simulink model "PMSM_FOC_ClosedLoop"  (R2025b)
settings: Solver=ode3  StartTime=0.0  StopTime=0.4  FixedStep=Ts_sim  RelTol=1e-3
PreLoadFcn:
  | params_pmsm_inverter
undefined symbols (not defined in the file or in its folder): Iq_max, J, Ki_curr, Ki_spd, Kp_curr, Kp_spd, Ld, Lq, pp, PsiPM, Rs, Ts_ctrl, Vdc, Vph_max
libraries: nesl_utility x13, fl_lib x9, ee_lib x8, slpidlib x3, simulink x2
(part 1 of 2)
settings Model: Creator=Harish  LastModifiedBy=Harish

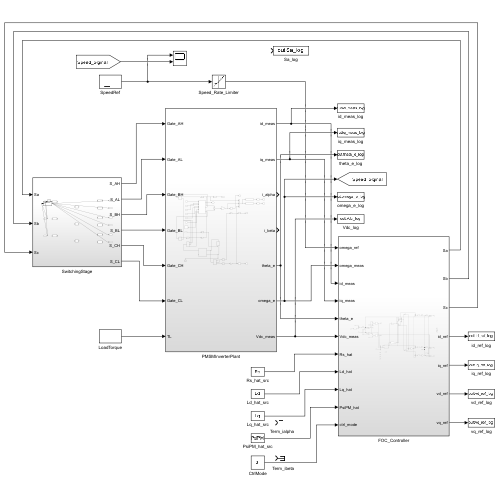
[thumbnail: Simulink's stored preview of the top-level diagram]
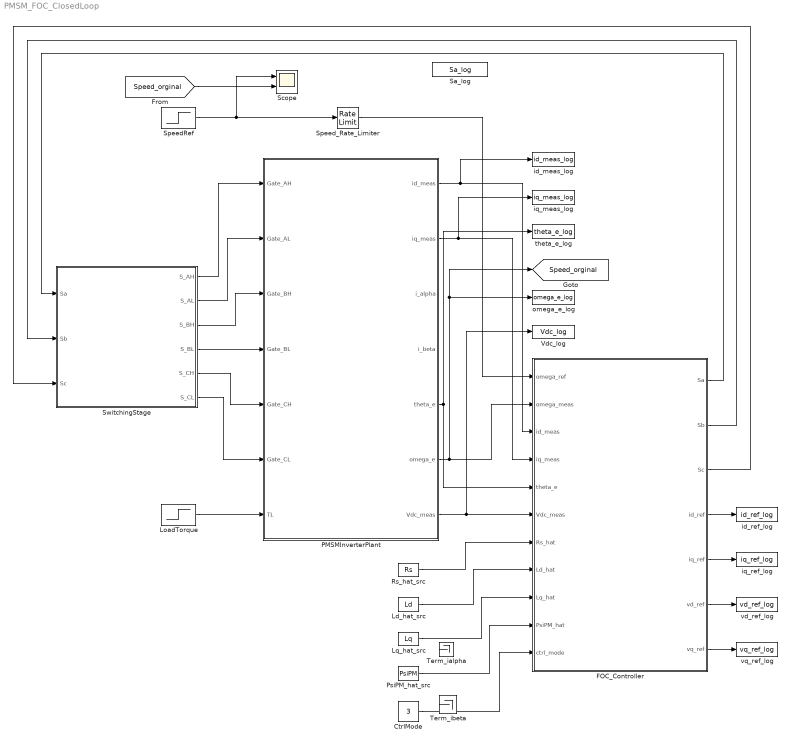
== system PMSM_FOC_ClosedLoop ==
  CtrlMode : Constant  Value=3
  FOC_Controller : Subsystem
  Ld_hat_src : Constant  Value=Ld
  LoadTorque : Step  Time=0.25  Before=0.0  After=0.05  SampleTime=0
  Lq_hat_src : Constant  Value=Lq
  PMSMInverterPlant : Subsystem
  PsiPM_hat_src : Constant  Value=PsiPM
  Rs_hat_src : Constant  Value=Rs
  Sa_log : ToWorkspace  VariableName=Sa_log  SaveFormat=Timeseries  SampleTime=-1
  Scope : Scope  NumInputPorts=2
      settings: ActiveDisplayYMinimum=-24.999999999999993  ActiveDisplayYMaximum=225
  SpeedRef : Step  Time=0.05  After=200  SampleTime=Ts_ctrl
  Speed_Rate_Limiter : RateLimiter  RisingSlewLimit=inf  FallingSlewLimit=-inf  SampleTimeMode=inherited
  SwitchingStage : Subsystem
  Term_ialpha : Terminator
  Term_ibeta : Terminator
  Vdc_log : ToWorkspace  VariableName=Vdc_log  SaveFormat=Timeseries  SampleTime=-1
  id_meas_log : ToWorkspace  VariableName=id_meas_log  SaveFormat=Timeseries  SampleTime=-1
  id_ref_log : ToWorkspace  VariableName=id_ref_log  SaveFormat=Timeseries  SampleTime=-1
  iq_meas_log : ToWorkspace  VariableName=iq_meas_log  SaveFormat=Timeseries  SampleTime=-1
  iq_ref_log : ToWorkspace  VariableName=iq_ref_log  SaveFormat=Timeseries  SampleTime=-1
  omega_e_log : ToWorkspace  VariableName=omega_e_log  SaveFormat=Timeseries  SampleTime=-1
  theta_e_log : ToWorkspace  VariableName=theta_e_log  SaveFormat=Timeseries  SampleTime=-1
  vd_ref_log : ToWorkspace  VariableName=vd_ref_log  SaveFormat=Timeseries  SampleTime=-1
  vq_ref_log : ToWorkspace  VariableName=vq_ref_log  SaveFormat=Timeseries  SampleTime=-1
  tag scope: Speed_orginal=global
  wires:
  [Speed_orginal] -> Scope/2
  SwitchingStage/5(S_CH) -> PMSMInverterPlant/5(Gate_CH)
  SwitchingStage/1(S_AH) -> PMSMInverterPlant/1(Gate_AH)
  SpeedRef/1 -> Scope/1, Speed_Rate_Limiter/1
  SwitchingStage/6(S_CL) -> PMSMInverterPlant/6(Gate_CL)
  FOC_Controller/2(Sb) -> SwitchingStage/2(Sb)
  PMSMInverterPlant/7(Vdc_meas) -> Vdc_log/1, FOC_Controller/6(Vdc_meas)
  SwitchingStage/2(S_AL) -> PMSMInverterPlant/2(Gate_AL)
  SwitchingStage/3(S_BH) -> PMSMInverterPlant/3(Gate_BH)
  PMSMInverterPlant/1(id_meas) -> FOC_Controller/3(id_meas), id_meas_log/1
  SwitchingStage/4(S_BL) -> PMSMInverterPlant/4(Gate_BL)
  LoadTorque/1 -> PMSMInverterPlant/7(TL)
  Speed_Rate_Limiter/1 -> FOC_Controller/1(omega_ref)
  FOC_Controller/3(Sc) -> SwitchingStage/3(Sc)
  PMSMInverterPlant/2(iq_meas) -> FOC_Controller/4(iq_meas), iq_meas_log/1
  PMSMInverterPlant/5(theta_e) -> FOC_Controller/5(theta_e), theta_e_log/1
  PMSMInverterPlant/6(omega_e) -> [Speed_orginal], omega_e_log/1, FOC_Controller/2(omega_meas)
  Rs_hat_src/1 -> FOC_Controller/7(Rs_hat)
  Ld_hat_src/1 -> FOC_Controller/8(Ld_hat)
  Lq_hat_src/1 -> FOC_Controller/9(Lq_hat)
  PsiPM_hat_src/1 -> FOC_Controller/10(PsiPM_hat)
  CtrlMode/1 -> FOC_Controller/11(ctrl_mode)
  FOC_Controller/1(Sa) -> SwitchingStage/1(Sa)
  FOC_Controller/4(id_ref) -> id_ref_log/1
  FOC_Controller/5(iq_ref) -> iq_ref_log/1
  FOC_Controller/6(vd_ref) -> vd_ref_log/1
  FOC_Controller/7(vq_ref) -> vq_ref_log/1

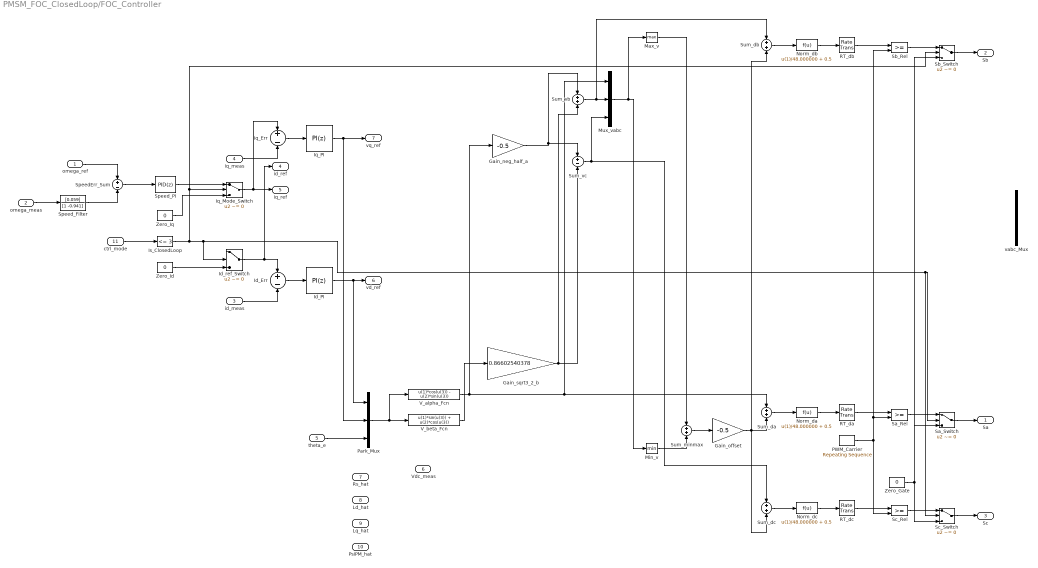
== system PMSM_FOC_ClosedLoop/FOC_Controller ==
  omega_ref : Inport  SampleTime=Ts_ctrl
  omega_meas : Inport  Port=2  SampleTime=Ts_ctrl
  id_meas : Inport  Port=3  SampleTime=Ts_ctrl
  iq_meas : Inport  Port=4  SampleTime=Ts_ctrl
  theta_e : Inport  Port=5  SampleTime=Ts_ctrl
  Vdc_meas : Inport  Port=6  SampleTime=Ts_ctrl
  Rs_hat : Inport  Port=7  SampleTime=Ts_ctrl
  Ld_hat : Inport  Port=8  SampleTime=Ts_ctrl
  Lq_hat : Inport  Port=9  SampleTime=Ts_ctrl
  PsiPM_hat : Inport  Port=10  SampleTime=Ts_ctrl
  ctrl_mode : Inport  Port=11  SampleTime=Ts_ctrl
  Gain_neg_half_a : Gain  Gain=-0.5
  Gain_offset : Gain  Gain=-0.5
  Gain_sqrt3_2_b : Gain  Gain=0.86602540378
  Id_Err : Sum  Inputs=+-
  Id_PI : slpidlib/PID Controller  Controller=PI  Form=Parallel  TimeDomain=Discrete-time  UseExternalTs=off  SampleTime=Ts_ctrl  IntegratorMethod=Forward Euler  FilterMethod=Forward Euler  ControllerParametersSource=internal  P=Kp_curr  I=Ki_curr  UseKiTs=off  D=0  UseExternalDerivativeSource=off  N=100  UseFilter=on  TunerSelectOption=Transfer Function Based (PID Tuner App)  InitialConditionSource=internal  InitialConditionForIntegrator=0  InitialConditionForFilter=0  DifferentiatorICPrevScaledInput=0  ExternalReset=none  TrackingMode=off  Kt=1  LimitOutput=on  SatLimitsSource=internal  UpperSaturationLimit=Vph_max  LowerSaturationLimit=-Vph_max  LinearizeAsGain=off  AntiWindupMode=clamping  Kb=1  LimitIntegrator=off  UpperIntegratorSaturationLimit=inf  LowerIntegratorSaturationLimit=-inf  POutMin=[]  POutMax=[]  IOutMin=[]  IOutMax=[]  DOutMin=[]  DOutMax=[]  NOutMin=[]  NOutMax=[]  SumOutMin=[]  SumOutMax=[]  SaturationOutMin=[]  SaturationOutMax=[]  PParamMin=[]  PParamMax=[]  IParamMin=[]  IParamMax=[]  DParamMin=[]  DParamMax=[]  NParamMin=[]  NParamMax=[]  KbParamMin=[]  KbParamMax=[]  KtParamMin=[]  KtParamMax=[]  KbOutMin=[]  KbOutMax=[]  KtOutMin=[]  KtOutMax=[]  IntegratorOutMin=[]  IntegratorOutMax=[]  FilterOutMin=[]  FilterOutMax=[]  SumI1OutMin=[]  SumI1OutMax=[]  SumI2OutMin=[]  SumI2OutMax=[]  SumI3OutMin=[]  SumI3OutMax=[]  SumI4OutMin=[]  SumI4OutMax=[]  SumDOutMin=[]  SumDOutMax=[]  DifferentiatorOutMin=[]  DifferentiatorOutMax=[]  FilterDiffOutCoefMin=[]  FilterDiffOutCoefMax=[]  ReciprocalOutMin=[]  ReciprocalOutMax=[]  SumDenOutMin=[]  SumDenOutMax=[]  SumNumOutMin=[]  SumNumOutMax=[]  DivideOutMin=[]  DivideOutMax=[]  UdiffTsProdOutMin=[]  UdiffTsProdOutMax=[]  NTsProdOutMin=[]  NTsProdOutMax=[]  UintegralTsProdOutMin=[]  UintegralTsProdOutMax=[]  UngainTsProdOutMin=[]  UngainTsProdOutMax=[]  ClampingZeroOutDataTypeStr=Inherit: Inherit via back propagation  ClampingZeroOutMin=[]  ClampingZeroOutMax=[]  FilterDenConstantOutDataTypeStr=Inherit: Inherit via back propagation  FilterDenConstantOutMin=[]  FilterDenConstantOutMax=[]  PCopyOutDataTypeStr=Inherit: Inherit via back propagation  PCopyOutMin=[]  PCopyOutMax=[]  NCopyOutDataTypeStr=Inherit: Inherit via back propagation  NCopyOutMin=[]  NCopyOutMax=[]  IntegratorContinuousStateAttributes=''  IntegratorStateMustResolveToSignalObject=off  IntegratorRTWStateStorageClass=Auto  FilterContinuousStateAttributes=''  FilterStateMustResolveToSignalObject=off  FilterRTWStateStorageClass=Auto  ParallelPVariant=InternalParameters  IdealPVariant=Disabled  IVariant=InternalParameters  DVariant=Disabled  IntegratorVariant=Discrete  SatVariant=Enabled  AWVariant=DiscClampingParallel  PCopyVariant=Disabled  TRVariant=Disabled  FdbkBlocksVariant=Forward  IdealPFdbkVariant=Disabled  SatFdbkVariant=Disabled  DerivativeFilterVariant=Disabled  NVariant=Disabled  NCopyVariant=Disabled_SignalSpec  FilterICVariant=Disabled  IntegratorICVariant=InternalICs  ExternalResetVariant=Disabled  TRSumVariant=Passthrough  SumFdbkVariant=Disabled  SumVariant=Sum_PI  TsampFilterVariant=InternalTs  TsampNgainVariant=Passthrough  TsampIntegralVariant=Disabled_SignalSpec  ExternalSaturationOutDataTypeStr=Inherit: Same as second input  DerivativeSourceVariant=Disabled  PreIntVariant=InternalPreInt
      settings: LibrarySourceBlock=simulink/Discrete/Discrete PID Controller
  Id_ref_Switch : Switch  Criteria=u2 ~= 0  SaturateOnIntegerOverflow=off  InputSameDT=off
  Iq_Err : Sum  Inputs=+-
  Iq_Mode_Switch : Switch  Criteria=u2 ~= 0  SaturateOnIntegerOverflow=off  InputSameDT=off
  Iq_PI : slpidlib/PID Controller  Controller=PI  Form=Parallel  TimeDomain=Discrete-time  UseExternalTs=off  SampleTime=Ts_ctrl  IntegratorMethod=Forward Euler  FilterMethod=Forward Euler  ControllerParametersSource=internal  P=Kp_curr  I=Ki_curr  UseKiTs=off  D=0  UseExternalDerivativeSource=off  N=100  UseFilter=on  TunerSelectOption=Transfer Function Based (PID Tuner App)  InitialConditionSource=internal  InitialConditionForIntegrator=0  InitialConditionForFilter=0  DifferentiatorICPrevScaledInput=0  ExternalReset=none  TrackingMode=off  Kt=1  LimitOutput=on  SatLimitsSource=internal  UpperSaturationLimit=Vph_max  LowerSaturationLimit=-Vph_max  LinearizeAsGain=off  AntiWindupMode=clamping  Kb=1  LimitIntegrator=off  UpperIntegratorSaturationLimit=inf  LowerIntegratorSaturationLimit=-inf  POutMin=[]  POutMax=[]  IOutMin=[]  IOutMax=[]  DOutMin=[]  DOutMax=[]  NOutMin=[]  NOutMax=[]  SumOutMin=[]  SumOutMax=[]  SaturationOutMin=[]  SaturationOutMax=[]  PParamMin=[]  PParamMax=[]  IParamMin=[]  IParamMax=[]  DParamMin=[]  DParamMax=[]  NParamMin=[]  NParamMax=[]  KbParamMin=[]  KbParamMax=[]  KtParamMin=[]  KtParamMax=[]  KbOutMin=[]  KbOutMax=[]  KtOutMin=[]  KtOutMax=[]  IntegratorOutMin=[]  IntegratorOutMax=[]  FilterOutMin=[]  FilterOutMax=[]  SumI1OutMin=[]  SumI1OutMax=[]  SumI2OutMin=[]  SumI2OutMax=[]  SumI3OutMin=[]  SumI3OutMax=[]  SumI4OutMin=[]  SumI4OutMax=[]  SumDOutMin=[]  SumDOutMax=[]  DifferentiatorOutMin=[]  DifferentiatorOutMax=[]  FilterDiffOutCoefMin=[]  FilterDiffOutCoefMax=[]  ReciprocalOutMin=[]  ReciprocalOutMax=[]  SumDenOutMin=[]  SumDenOutMax=[]  SumNumOutMin=[]  SumNumOutMax=[]  DivideOutMin=[]  DivideOutMax=[]  UdiffTsProdOutMin=[]  UdiffTsProdOutMax=[]  NTsProdOutMin=[]  NTsProdOutMax=[]  UintegralTsProdOutMin=[]  UintegralTsProdOutMax=[]  UngainTsProdOutMin=[]  UngainTsProdOutMax=[]  ClampingZeroOutDataTypeStr=Inherit: Inherit via back propagation  ClampingZeroOutMin=[]  ClampingZeroOutMax=[]  FilterDenConstantOutDataTypeStr=Inherit: Inherit via back propagation  FilterDenConstantOutMin=[]  FilterDenConstantOutMax=[]  PCopyOutDataTypeStr=Inherit: Inherit via back propagation  PCopyOutMin=[]  PCopyOutMax=[]  NCopyOutDataTypeStr=Inherit: Inherit via back propagation  NCopyOutMin=[]  NCopyOutMax=[]  IntegratorContinuousStateAttributes=''  IntegratorStateMustResolveToSignalObject=off  IntegratorRTWStateStorageClass=Auto  FilterContinuousStateAttributes=''  FilterStateMustResolveToSignalObject=off  FilterRTWStateStorageClass=Auto  ParallelPVariant=InternalParameters  IdealPVariant=Disabled  IVariant=InternalParameters  DVariant=Disabled  IntegratorVariant=Discrete  SatVariant=Enabled  AWVariant=DiscClampingParallel  PCopyVariant=Disabled  TRVariant=Disabled  FdbkBlocksVariant=Forward  IdealPFdbkVariant=Disabled  SatFdbkVariant=Disabled  DerivativeFilterVariant=Disabled  NVariant=Disabled  NCopyVariant=Disabled_SignalSpec  FilterICVariant=Disabled  IntegratorICVariant=InternalICs  ExternalResetVariant=Disabled  TRSumVariant=Passthrough  SumFdbkVariant=Disabled  SumVariant=Sum_PI  TsampFilterVariant=InternalTs  TsampNgainVariant=Passthrough  TsampIntegralVariant=Disabled_SignalSpec  ExternalSaturationOutDataTypeStr=Inherit: Same as second input  DerivativeSourceVariant=Disabled  PreIntVariant=InternalPreInt
      settings: LibrarySourceBlock=simulink/Discrete/Discrete PID Controller
  Is_ClosedLoop : simulink/Logic and Bit Operations/Compare To Constant  relop=<=  const=3  OutDataTypeStr=boolean
  Max_v : MinMax  Function=max
  Min_v : MinMax
  Mux_vabc : Mux  Inputs=3
  Norm_da : Fcn  Expr=u(1)/48.000000 + 0.5
  Norm_db : Fcn  Expr=u(1)/48.000000 + 0.5
  Norm_dc : Fcn  Expr=u(1)/48.000000 + 0.5
  PWM_Carrier : simulink/Sources/Repeating Sequence  rep_seq_t=[0, Ts_ctrl/2, Ts_ctrl]  rep_seq_y=[0, 1, 0]
  Park_Mux : Mux  Inputs=3
  RT_da : RateTransition  OutPortSampleTime=Ts_sim
  RT_db : RateTransition  OutPortSampleTime=Ts_sim
  RT_dc : RateTransition  OutPortSampleTime=Ts_sim
  Sa_Rel : RelationalOperator  OutDataTypeStr=boolean  RndMeth=Simplest  InputSameDT=off
  Sa_Switch : Switch  Criteria=u2 ~= 0  SaturateOnIntegerOverflow=off  InputSameDT=off
  Sb_Rel : RelationalOperator  OutDataTypeStr=boolean  RndMeth=Simplest  InputSameDT=off
  Sb_Switch : Switch  Criteria=u2 ~= 0  SaturateOnIntegerOverflow=off  InputSameDT=off
  Sc_Rel : RelationalOperator  OutDataTypeStr=boolean  RndMeth=Simplest  InputSameDT=off
  Sc_Switch : Switch  Criteria=u2 ~= 0  SaturateOnIntegerOverflow=off  InputSameDT=off
  SpeedErr_Sum : Sum  Inputs=+-
  Speed_Filter : DiscreteFilter  Numerator=[0.059]  Denominator=[1 -0.941]  SampleTime=Ts_ctrl
  Speed_PI : slpidlib/PID Controller  Controller=PID  Form=Parallel  TimeDomain=Discrete-time  UseExternalTs=off  SampleTime=Ts_ctrl  IntegratorMethod=Forward Euler  FilterMethod=Forward Euler  ControllerParametersSource=internal  P=Kp_spd  I=Ki_spd  UseKiTs=off  D=0  UseExternalDerivativeSource=off  N=100  UseFilter=on  TunerSelectOption=Transfer Function Based (PID Tuner App)  InitialConditionSource=internal  InitialConditionForIntegrator=0  InitialConditionForFilter=0  DifferentiatorICPrevScaledInput=0  ExternalReset=none  TrackingMode=off  Kt=1  LimitOutput=on  SatLimitsSource=internal  UpperSaturationLimit=Iq_max  LowerSaturationLimit=-Iq_max  LinearizeAsGain=on  AntiWindupMode=clamping  Kb=1  LimitIntegrator=off  UpperIntegratorSaturationLimit=inf  LowerIntegratorSaturationLimit=-inf  POutMin=[]  POutMax=[]  IOutMin=[]  IOutMax=[]  DOutMin=[]  DOutMax=[]  NOutMin=[]  NOutMax=[]  SumOutMin=[]  SumOutMax=[]  SaturationOutMin=[]  SaturationOutMax=[]  PParamMin=[]  PParamMax=[]  IParamMin=[]  IParamMax=[]  DParamMin=[]  DParamMax=[]  NParamMin=[]  NParamMax=[]  KbParamMin=[]  KbParamMax=[]  KtParamMin=[]  KtParamMax=[]  KbOutMin=[]  KbOutMax=[]  KtOutMin=[]  KtOutMax=[]  IntegratorOutMin=[]  IntegratorOutMax=[]  FilterOutMin=[]  FilterOutMax=[]  SumI1OutMin=[]  SumI1OutMax=[]  SumI2OutMin=[]  SumI2OutMax=[]  SumI3OutMin=[]  SumI3OutMax=[]  SumI4OutMin=[]  SumI4OutMax=[]  SumDOutMin=[]  SumDOutMax=[]  DifferentiatorOutMin=[]  DifferentiatorOutMax=[]  FilterDiffOutCoefMin=[]  FilterDiffOutCoefMax=[]  ReciprocalOutMin=[]  ReciprocalOutMax=[]  SumDenOutMin=[]  SumDenOutMax=[]  SumNumOutMin=[]  SumNumOutMax=[]  DivideOutMin=[]  DivideOutMax=[]  UdiffTsProdOutMin=[]  UdiffTsProdOutMax=[]  NTsProdOutMin=[]  NTsProdOutMax=[]  UintegralTsProdOutMin=[]  UintegralTsProdOutMax=[]  UngainTsProdOutMin=[]  UngainTsProdOutMax=[]  ClampingZeroOutDataTypeStr=Inherit: Inherit via back propagation  ClampingZeroOutMin=[]  ClampingZeroOutMax=[]  FilterDenConstantOutDataTypeStr=Inherit: Inherit via back propagation  FilterDenConstantOutMin=[]  FilterDenConstantOutMax=[]  PCopyOutDataTypeStr=Inherit: Inherit via back propagation  PCopyOutMin=[]  PCopyOutMax=[]  NCopyOutDataTypeStr=Inherit: Inherit via back propagation  NCopyOutMin=[]  NCopyOutMax=[]  IntegratorContinuousStateAttributes=''  IntegratorStateMustResolveToSignalObject=off  IntegratorRTWStateStorageClass=Auto  FilterContinuousStateAttributes=''  FilterStateMustResolveToSignalObject=off  FilterRTWStateStorageClass=Auto  ParallelPVariant=InternalParameters  IdealPVariant=Disabled  IVariant=InternalParameters  DVariant=InternalParameters  IntegratorVariant=Discrete  SatVariant=Enabled  AWVariant=DiscClampingParallel  PCopyVariant=Disabled  TRVariant=Disabled  FdbkBlocksVariant=Forward  IdealPFdbkVariant=Disabled  SatFdbkVariant=Disabled  DerivativeFilterVariant=ForwardEulerFilter  NVariant=InternalParameters  NCopyVariant=Disabled  FilterICVariant=InternalICsFilter  IntegratorICVariant=InternalICs  ExternalResetVariant=Disabled  TRSumVariant=Passthrough  SumFdbkVariant=Disabled  SumVariant=Sum_PID  TsampFilterVariant=InternalTs  TsampNgainVariant=Passthrough  TsampIntegralVariant=Disabled_SignalSpec  ExternalSaturationOutDataTypeStr=Inherit: Same as second input  DerivativeSourceVariant=ErrorSignal  PreIntVariant=InternalPreInt
  Sum_da : Sum
  Sum_db : Sum
  Sum_dc : Sum
  Sum_minmax : Sum
  Sum_vb : Sum
  Sum_vc : Sum  Inputs=+-
  V_alpha_Fcn : Fcn  Expr=u(1)*cos(u(3)) - u(2)*sin(u(3))
  V_beta_Fcn : Fcn  Expr=u(1)*sin(u(3)) + u(2)*cos(u(3))
  Zero_Gate : Constant  Value=0  OutDataTypeStr=boolean  SampleTime=Ts_ctrl
  Zero_Id : Constant  Value=0
  Zero_Iq : Constant  Value=0  SampleTime=Ts_ctrl
  vabc_Mux : Mux  Inputs=3
  Sa : Outport
  Sb : Outport  Port=2
  Sc : Outport  Port=3
  id_ref : Outport  Port=4  SampleTime=Ts_ctrl
  iq_ref : Outport  Port=5  SampleTime=Ts_ctrl
  vd_ref : Outport  Port=6  SampleTime=Ts_ctrl
  vq_ref : Outport  Port=7  SampleTime=Ts_ctrl
  wires:
  Speed_PI/1 -> Iq_Mode_Switch/1
  Zero_Id/1 -> Id_ref_Switch/3
  omega_meas/1 -> Speed_Filter/1
  Is_ClosedLoop/1 -> Sc_Switch/2, Sa_Switch/2, Id_ref_Switch/2, Iq_Mode_Switch/2, Sb_Switch/2
  ctrl_mode/1 -> Is_ClosedLoop/1
  Zero_Iq/1 -> Iq_Mode_Switch/3
  Id_Err/1 -> Id_PI/1
  omega_ref/1 -> SpeedErr_Sum/1
  Speed_Filter/1 -> SpeedErr_Sum/2
  Zero_Gate/1 -> Sb_Switch/3, Sc_Switch/3, Sa_Switch/3
  SpeedErr_Sum/1 -> Speed_PI/1
  iq_meas/1 -> Iq_Err/2
  Iq_Mode_Switch/1 -> Iq_Err/1, iq_ref/1
  theta_e/1 -> Park_Mux/3
  Id_ref_Switch/1 -> Id_Err/1, id_ref/1
  id_meas/1 -> Id_Err/2
  Iq_Err/1 -> Iq_PI/1
  Sb_Rel/1 -> Sb_Switch/1
  Sum_db/1 -> Norm_db/1
  Iq_PI/1 -> Park_Mux/2, vq_ref/1
  Sb_Switch/1 -> Sb/1
  Gain_neg_half_a/1 -> Sum_vc/1, Sum_vb/1
  Id_PI/1 -> Park_Mux/1, vd_ref/1
  Norm_dc/1 -> RT_dc/1
  Park_Mux/1 -> V_alpha_Fcn/1, V_beta_Fcn/1
  Sa_Switch/1 -> Sa/1
  Sum_da/1 -> Norm_da/1
  V_alpha_Fcn/1 -> Sum_da/1, Mux_vabc/1, Gain_neg_half_a/1
  Gain_offset/1 -> Sum_da/2, Sum_db/2, Sum_dc/2
  V_beta_Fcn/1 -> Gain_sqrt3_2_b/1
  Gain_sqrt3_2_b/1 -> Sum_vb/2, Sum_vc/2
  Min_v/1 -> Sum_minmax/2
  Sum_vb/1 -> Sum_db/1, Mux_vabc/2
  Sum_dc/1 -> Norm_dc/1
  Sum_vc/1 -> Sum_dc/1, Mux_vabc/3
  Mux_vabc/1 -> Max_v/1, Min_v/1
  Max_v/1 -> Sum_minmax/1
  Sum_minmax/1 -> Gain_offset/1
  Norm_db/1 -> RT_db/1
  Norm_da/1 -> RT_da/1
  RT_db/1 -> Sb_Rel/1
  RT_da/1 -> Sa_Rel/1
  PWM_Carrier/1 -> Sb_Rel/2, Sa_Rel/2, Sc_Rel/2
  Sc_Switch/1 -> Sc/1
  RT_dc/1 -> Sc_Rel/1
  Sa_Rel/1 -> Sa_Switch/1
  Sc_Rel/1 -> Sc_Switch/1

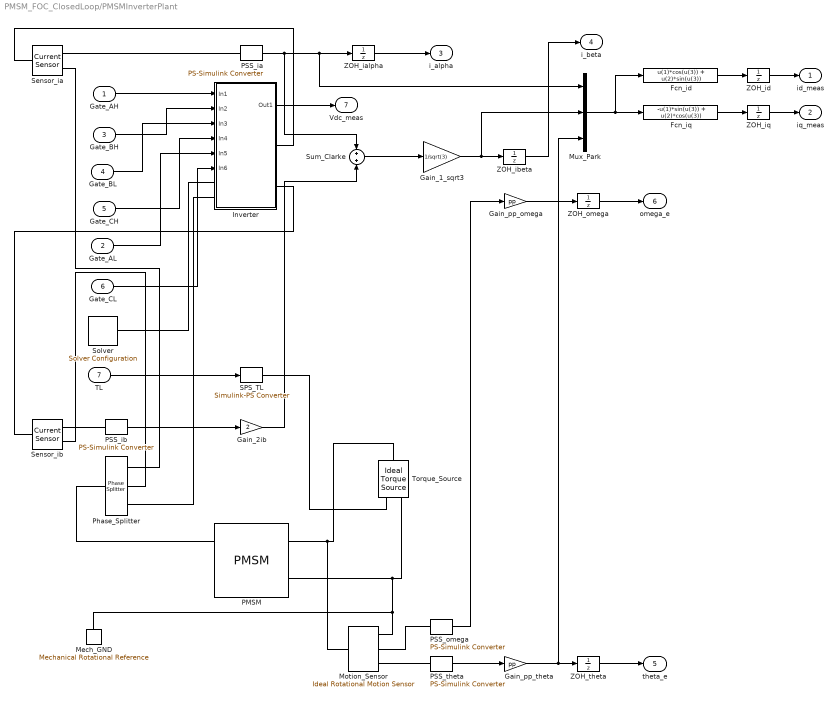
== system PMSM_FOC_ClosedLoop/PMSMInverterPlant ==
  Gate_AH : Inport
  Gate_AL : Inport  Port=2
  Gate_BH : Inport  Port=3
  Gate_BL : Inport  Port=4
  Gate_CH : Inport  Port=5
  Gate_CL : Inport  Port=6
  TL : Inport  Port=7
  Fcn_id : Fcn  Expr=u(1)*cos(u(3)) + u(2)*sin(u(3))
  Fcn_iq : Fcn  Expr=-u(1)*sin(u(3)) + u(2)*cos(u(3))
  Gain_1_sqrt3 : Gain  Gain=1/sqrt(3)
  Gain_2ib : Gain  Gain=2
  Gain_pp_omega : Gain  Gain=pp
  Gain_pp_theta : Gain  Gain=pp
  Inverter : Subsystem
  Mech_GND : fl_lib/Mechanical/Rotational Elements/Mechanical Rotational Reference
  Motion_Sensor : fl_lib/Mechanical/Mechanical Sensors/Ideal Rotational Motion Sensor  reference=foundation.enum.MeasurementReference.difference  acceleration_port=false  velocity_port=true  position_port=true  wrap_angle=false  offset=0 rad
  Mux_Park : Mux  Inputs=3
  PMSM : ee_lib/Electromechanical/Permanent Magnet/PMSM  port_option=1  winding_type=ee.enum.electromech.statorconfiguration.wye  machine_param=ee.enum.pmsm.parameterization.constant  nPolePairs=pp  pmflux_param=ee.enum.pmflux.fluxlinkage  pm_flux_linkage=PsiPM Wb  torque_constant=0.18 N*m/A  back_emf_constant=0.18 V*s/rad  stator_param=1  Ld=Ld H  Lq=Lq H  idVec=[-200, 0, 200] A  iqVec=[-200, 0, 200] A  LdMatrix=0.0002 * ones(3, 3) H  LqMatrix=0.0002 * ones(3, 3) H  PmMatrix=0.1 * ones(3, 3) Wb  ktMatrix=0.18 * ones(3, 3) N*m/A  keMatrix=0.18 * ones(3, 3) V*s/rad  L0=0.00016 H  Ls=0.0002 H  Lm=-0.00002 H  Ms=0.00002 H  Rs=Rs Ohm  zero_sequence=ee.enum.park.zerosequence.include  axes_param=ee.enum.rotorangle.daxis  loss_param=ee.enum.ironloss.none  losses_oc=[0, 0, 0] W  losses_sc=[0, 0, 0] W  f_losses=60 Hz  Isc_losses=95 A  J=J kg*m^2  lam=B_fric N*m*s/rad  i_d_specify=off  i_d_priority=None  i_d=0 A  i_d_nominal_specify=off  i_d_nominal_value=1  i_d_nominal_unit=A  i_q_specify=off  i_q_priority=None  i_q=0 A  i_q_nominal_specify=off  i_q_nominal_value=1  i_q_nominal_unit=A  torque_specify=off  torque_priority=None  torque=0 N*m  torque_nominal_specify=off  torque_nominal_value=1  torque_nominal_unit=N*m  angular_velocity_specify=off  angular_velocity_priority=High  angular_velocity=0 rpm  angular_velocity_nominal_specify=off  angular_velocity_nominal_value=1  angular_velocity_nominal_unit=rpm  angular_position_specify=off  angular_position_priority=High  angular_position=0 deg  angular_position_nominal_specify=off  angular_position_nominal_value=1  angular_position_nominal_unit=deg  alpha=3.93e-3 1/K  alpha_flux=-0.001 1/K  Tmeas=298.15 K  stator_thermal_mass=100 J/K  rotor_thermal_mass=200 J/K  Rm_percent_rotor=90  Rd_percent_rotor=30  temperatureA_specify=off  temperatureA_priority=High  temperatureA=25 degC  temperatureA_nominal_specify=off  temperatureA_nominal_value=1  temperatureA_nominal_unit=degC  temperatureB_specify=off  temperatureB_priority=High  temperatureB=25 degC  temperatureB_nominal_specify=off  temperatureB_nominal_value=1  temperatureB_nominal_unit=degC  temperatureC_specify=off  temperatureC_priority=High  temperatureC=25 degC  temperatureC_nominal_specify=off  temperatureC_nominal_value=1  temperatureC_nominal_unit=degC  temperatureR_specify=off  temperatureR_priority=High  temperatureR=25 degC  temperatureR_nominal_specify=off  temperatureR_nominal_value=1  temperatureR_nominal_unit=degC
      settings: InternalSimscapePortConfiguration="{\"Bottom\":[],\"Left\":[{\"id\":\"N\",\"label\":\"~\",\"type\":\"foundation.electrical.three_phase\"},{\"id\":\"n\",\"label\":\"n\",\"type\":\"foundation.electrical.electrical\"}],\"Right\":[{\"id\":\"R\",\"label\":\"R\",\"type\":\"foundation.mechanical.rotational.rotational\"},{\"id\":\"C\",\"label\":\"C\",\"type\":\"foundation.mechanical.rotational.rotational\"}],\"Top\":[]}"
  PSS_ia : nesl_utility/PS-Simulink Converter  PhysicalDomain=network_engine_domain  SubClassName=ps_output  LeftPortType=input  RightPortType=output  PseudoPeriodic=off  Frequencies=[]  VectorFormat=inherit  Unit=inherit  AffineConversion=off
  PSS_ib : nesl_utility/PS-Simulink Converter  PhysicalDomain=network_engine_domain  SubClassName=ps_output  LeftPortType=input  RightPortType=output  PseudoPeriodic=off  Frequencies=[]  VectorFormat=inherit  Unit=inherit  AffineConversion=off
  PSS_omega : nesl_utility/PS-Simulink Converter  PhysicalDomain=network_engine_domain  SubClassName=ps_output  LeftPortType=input  RightPortType=output  PseudoPeriodic=off  Frequencies=[]  VectorFormat=inherit  Unit=inherit  AffineConversion=off
  PSS_theta : nesl_utility/PS-Simulink Converter  PhysicalDomain=network_engine_domain  SubClassName=ps_output  LeftPortType=input  RightPortType=output  PseudoPeriodic=off  Frequencies=[]  VectorFormat=inherit  Unit=inherit  AffineConversion=off
  Phase_Splitter : ee_lib/Connectors & References/Phase Splitter
  SPS_TL : nesl_utility/Simulink-PS Converter  PhysicalDomain=network_engine_domain  SubClassName=ps_input  LeftPortType=input  RightPortType=output  PseudoPeriodic=off  Frequencies=[]  NoiseDistribution=none  NoiseParameters=[]  Unit=1  AffineConversion=off  FilteringAndDerivatives=filter  SimscapeFilterOrder=1  InputFilterTimeConstant=0.001  UdotUserProvided=0
  Sensor_ia : fl_lib/Electrical/Electrical Sensors/Current Sensor
  Sensor_ib : fl_lib/Electrical/Electrical Sensors/Current Sensor
  Solver : nesl_utility/Solver Configuration  PhysicalDomain=network_engine_domain  SubClassName=solver  LeftPortType=input  RightPortType=generic  Tones=[]  Harmonics=[]  SimulateNoise=off  Profile=off  UseLocalSampling=off  EnableSwitchedLinearOptims=on  FrequencyDomain=off  UseCCode=off  RelTol=0.001  AbsTol=0.001  MinStep=1e-09  ToWorkspace=off  RevertToSquareIcSolve=off  NumHomotopyIterations=100  PhasorMode=off  PhasorModeNumHarmonics=1  ConsistencySolver=NEWTON_XTOL_AFTER_FTOL  IndexReductionMethod=DerivativeReplacement  DoDC=off  ResidualTolerance=1e-09  ConsistencyTolSource=GLOBAL  ConsistencyAbsTol=0.001  ConsistencyRelTol=0.001  ConsistencyTolFactor=0.001  UseLocalSolver=on  LocalSolverChoice=NE_BACKWARD_EULER_ADVANCER  ResolveIndetEquations=on  FunctionEvalNumThread=1  LocalSolverSampleTime=Ts_sim  DoFixedCost=off  MaxNonlinIter=3  MaxModeIter=2  ComputeImpulses=off  ImpulseIterations=2  LinearAlgebra=auto  LinearAlgebraNumThread=0  EquationFormulation=NE_TIME_EF  DelaysMemoryBudget=1024  AutomaticFiltering=on  FilteringTimeConstant=0.001  PartitionStorageMethod=AS_NEEDED  PartitionMemoryBudget=1024  PartitionMethod=ROBUST  MultibodyUseLocalSolver=off  MultibodyLocalSolverChoice=ODE1  MultibodyLocalSolverSampleTime=0.001
  Sum_Clarke : Sum
  Torque_Source : fl_lib/Mechanical/Mechanical Sources/Ideal Torque Source
  ZOH_ialpha : UnitDelay  SampleTime=Ts_ctrl  HasFrameUpgradeWarning=on
  ZOH_ibeta : UnitDelay  SampleTime=Ts_ctrl  HasFrameUpgradeWarning=on
  ZOH_id : UnitDelay  SampleTime=Ts_ctrl  HasFrameUpgradeWarning=on
  ZOH_iq : UnitDelay  SampleTime=Ts_ctrl  HasFrameUpgradeWarning=on
  ZOH_omega : UnitDelay  SampleTime=Ts_ctrl  HasFrameUpgradeWarning=on
  ZOH_theta : UnitDelay  SampleTime=Ts_ctrl  HasFrameUpgradeWarning=on
  id_meas : Outport
  iq_meas : Outport  Port=2
  i_alpha : Outport  Port=3
  i_beta : Outport  Port=4
  theta_e : Outport  Port=5
  omega_e : Outport  Port=6
  Vdc_meas : Outport  Port=7
  wires:
  Mux_Park/1 -> Fcn_id/1, Fcn_iq/1
  Gain_1_sqrt3/1 -> Mux_Park/2, ZOH_ibeta/1
  Gate_AH/1 -> Inverter/1(In1)
  ZOH_ibeta/1 -> i_beta/1
  Gate_CH/1 -> Inverter/4(In4)
  Fcn_id/1 -> ZOH_id/1
  Gate_BH/1 -> Inverter/2(In2)
  Gate_BL/1 -> Inverter/3(In3)
  Gate_AL/1 -> Inverter/5(In5)
  Gate_CL/1 -> Inverter/6(In6)
  TL/1 -> SPS_TL/1
  PSS_ib/1 -> Gain_2ib/1
  Gain_pp_omega/1 -> ZOH_omega/1
  PSS_ia/1 -> Mux_Park/1, ZOH_ialpha/1, Sum_Clarke/1
  ZOH_id/1 -> id_meas/1
  Inverter/1(Out1) -> Vdc_meas/1
  Gain_2ib/1 -> Sum_Clarke/2
  ZOH_ialpha/1 -> i_alpha/1
  Sum_Clarke/1 -> Gain_1_sqrt3/1
  PSS_omega/1 -> Gain_pp_omega/1
  PSS_theta/1 -> Gain_pp_theta/1
  Gain_pp_theta/1 -> Mux_Park/3, ZOH_theta/1
  ZOH_omega/1 -> omega_e/1
  ZOH_theta/1 -> theta_e/1
  Fcn_iq/1 -> ZOH_iq/1
  ZOH_iq/1 -> iq_meas/1
  connections:
  Sensor_ib/RConn1 -- PSS_ib/LConn1
  Sensor_ia/RConn1 -- PSS_ia/LConn1
  Motion_Sensor/RConn2 -- PSS_omega/LConn1
  Sensor_ib/RConn2 -- Phase_Splitter/RConn2
  Sensor_ia/RConn2 -- Phase_Splitter/RConn1
  Inverter/RConn2 -- Sensor_ib/LConn1
  Phase_Splitter/LConn1 -- PMSM/LConn1
  Solver/RConn1 -- Inverter/LConn1
  Phase_Splitter/RConn3 -- Inverter/LConn2
  Mech_GND/LConn1 -- PMSM/RConn2 -- Torque_Source/RConn2 -- Motion_Sensor/RConn1
  Inverter/RConn1 -- Sensor_ia/LConn1
  SPS_TL/RConn1 -- Torque_Source/RConn1
  PMSM/RConn1 -- Torque_Source/LConn1 -- Motion_Sensor/LConn1
  Motion_Sensor/RConn3 -- PSS_theta/LConn1

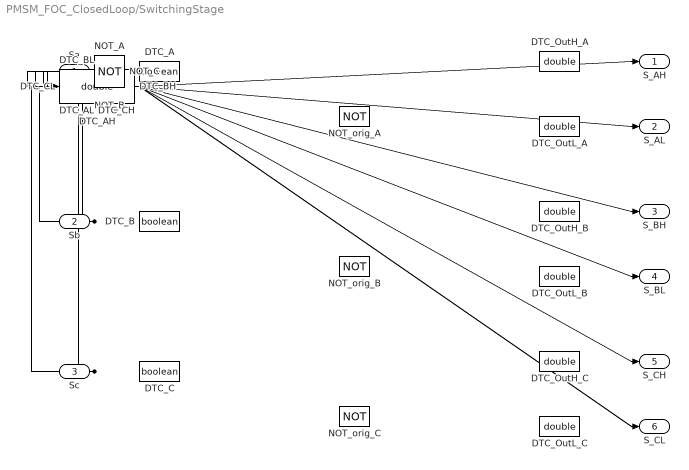
== system PMSM_FOC_ClosedLoop/SwitchingStage ==
  Sa : Inport
  Sb : Inport  Port=2
  Sc : Inport  Port=3
  DTC_A : DataTypeConversion  OutDataTypeStr=boolean  SaturateOnIntegerOverflow=off  RndMeth=Floor
  DTC_AH : DataTypeConversion  OutDataTypeStr=double  SaturateOnIntegerOverflow=off  RndMeth=Floor
  DTC_AL : DataTypeConversion  OutDataTypeStr=double  SaturateOnIntegerOverflow=off  RndMeth=Floor
  DTC_B : DataTypeConversion  OutDataTypeStr=boolean  SaturateOnIntegerOverflow=off  RndMeth=Floor
  DTC_BH : DataTypeConversion  OutDataTypeStr=double  SaturateOnIntegerOverflow=off  RndMeth=Floor
  DTC_BL : DataTypeConversion  OutDataTypeStr=double  SaturateOnIntegerOverflow=off  RndMeth=Floor
  DTC_C : DataTypeConversion  OutDataTypeStr=boolean  SaturateOnIntegerOverflow=off  RndMeth=Floor
  DTC_CH : DataTypeConversion  OutDataTypeStr=double  SaturateOnIntegerOverflow=off  RndMeth=Floor
  DTC_CL : DataTypeConversion  OutDataTypeStr=double  SaturateOnIntegerOverflow=off  RndMeth=Floor
  DTC_OutH_A : DataTypeConversion  OutDataTypeStr=double  SaturateOnIntegerOverflow=off  RndMeth=Floor
  DTC_OutH_B : DataTypeConversion  OutDataTypeStr=double  SaturateOnIntegerOverflow=off  RndMeth=Floor
  DTC_OutH_C : DataTypeConversion  OutDataTypeStr=double  SaturateOnIntegerOverflow=off  RndMeth=Floor
  DTC_OutL_A : DataTypeConversion  OutDataTypeStr=double  SaturateOnIntegerOverflow=off  RndMeth=Floor
  DTC_OutL_B : DataTypeConversion  OutDataTypeStr=double  SaturateOnIntegerOverflow=off  RndMeth=Floor
  DTC_OutL_C : DataTypeConversion  OutDataTypeStr=double  SaturateOnIntegerOverflow=off  RndMeth=Floor
  NOT_A : Logic  Operator=NOT  AllPortsSameDT=off  OutDataTypeStr=boolean
  NOT_B : Logic  Operator=NOT  AllPortsSameDT=off  OutDataTypeStr=boolean
  NOT_C : Logic  Operator=NOT  AllPortsSameDT=off  OutDataTypeStr=boolean
  NOT_orig_A : Logic  Operator=NOT  AllPortsSameDT=off  OutDataTypeStr=boolean
  NOT_orig_B : Logic  Operator=NOT  AllPortsSameDT=off  OutDataTypeStr=boolean
  NOT_orig_C : Logic  Operator=NOT  AllPortsSameDT=off  OutDataTypeStr=boolean
  S_AH : Outport
  S_AL : Outport  Port=2
  S_BH : Outport  Port=3
  S_BL : Outport  Port=4
  S_CH : Outport  Port=5
  S_CL : Outport  Port=6
  wires:
  Sa/1 -> DTC_AH/1, NOT_A/1
  DTC_AH/1 -> S_AH/1
  NOT_A/1 -> DTC_AL/1
  DTC_AL/1 -> S_AL/1
  Sb/1 -> DTC_BH/1, NOT_B/1
  DTC_BH/1 -> S_BH/1
  NOT_B/1 -> DTC_BL/1
  DTC_BL/1 -> S_BL/1
  Sc/1 -> DTC_CH/1, NOT_C/1
  DTC_CH/1 -> S_CH/1
  NOT_C/1 -> DTC_CL/1
  DTC_CL/1 -> S_CL/1
